simulink model "Lab1_Water_Tank_Level_Calibrated"  (R2017b)
settings: Solver=VariableStepAuto  StartTime=0.0  StopTime=60  RelTol=1e-3
settings Model: Creator=beena  LastModifiedBy=Joseph

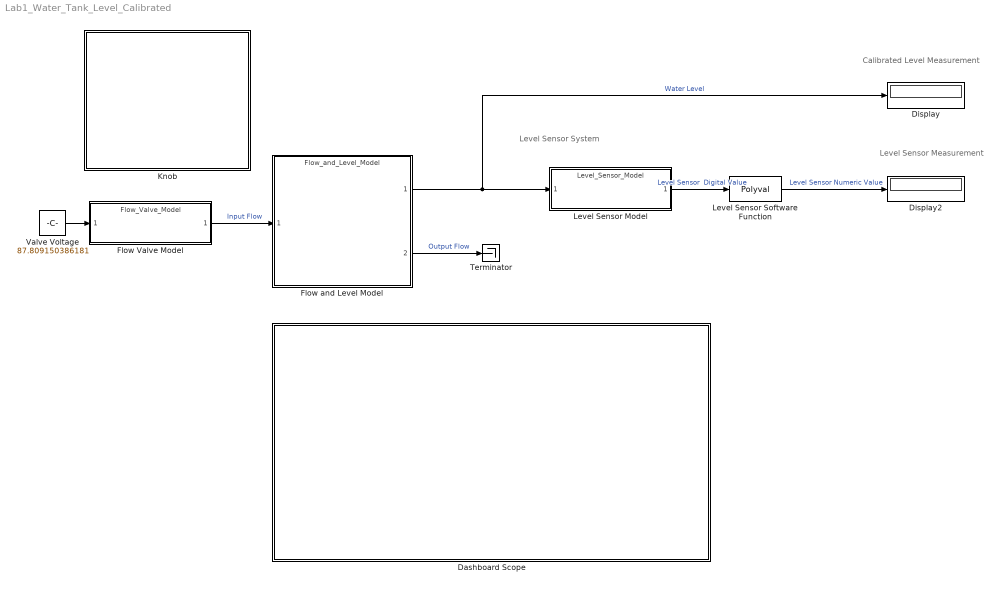
== system Lab1_Water_Tank_Level_Calibrated ==
  note: Level Sensor System
  note: Calibrated Level Measurement
  note: Level Sensor Measurement
  Dashboard Scope : Subsystem  DialogController=hmiCreateDDGDialog  IsWebBlock=on  mask(MWDashboardBlock){webBlockId=2a1a89e9-3606-4793-9b6e-01017e02ca12, webBlockType=sdiscope, ShowInitialText=on, HMISrcModelName=Lab1_Water_Tank_Level_Calibrated}
      mask prompts: webBlockId "WebBlock Id"; webBlockType "WebBlock Type"; HMISrcModelName "Source Model"
      mask help: SimulinkHMI:dialogs:HMIScopeDialogDesc
      mask Help: helpview([docroot '/mapfiles/simulink.map'], 'hmi_scope')
      mask Display:
      | if strcmp(get_param(bdroot(gcb),'BlockDiagramType'), 'library')
      |     image([(matlabroot) '/toolbox/simulink/hmi/icons/DashboardScope.png']);
      | end
  Display : Display
  Display2 : Display
  Flow Valve Model : ModelReference  ModelNameDialog=Flow_Valve_Model.slxp  ModelReferenceVersion=1.41  CopyOfModelProtected=on
  Flow and Level Model : ModelReference  ModelNameDialog=Flow_and_Level_Model.slxp  ModelReferenceVersion=1.41  CopyOfModelProtected=on
  Knob : Subsystem  DialogController=hmiCreateDDGDialog  IsWebBlock=on  mask(MWDashboardBlock){webBlockId=f1d15619-c2b9-4264-80fc-b36746c0ed4a, webBlockType=continuousknob, ShowInLibBrowser=on, ShowInitialText=on, HMISrcModelName=Lab1_Water_Tank_Level_Calibrated}
      mask prompts: webBlockId "WebBlock Id"; webBlockType "WebBlock Type"; HMISrcModelName "Source Model"
      mask help: SimulinkHMI:dialogs:ContinuousKnobDialogDesc
      mask Help: helpview([docroot '/mapfiles/simulink.map'], 'hmi_knob')
      mask Display:
      | if strcmp(get_param(bdroot(gcb),'BlockDiagramType'), 'library')
      |     image([(matlabroot) '/toolbox/simulink/hmi/icons/ContinuousKnob.png']);
      | end
  Level Sensor Software Function : Polyval  Coefs="[0.2001    0.0005]"
  Level Sensor Model : ModelReference  ModelNameDialog=Level_Sensor_Model.slxp  ModelReferenceVersion=1.51  CopyOfModelProtected=on
  Terminator : Terminator
  Valve Voltage : Constant  Value=87.809150386181
  wires:
  Flow and Level Model/1 -> Level Sensor Model/1, Display/1  "Water Level"
  Flow and Level Model/2 -> Terminator/1  "Output Flow"
  Flow Valve Model/1 -> Flow and Level Model/1  "Input Flow"
  Level Sensor Model/1 -> Level Sensor Software Function/1  "Level Sensor  Digital Value"
  Level Sensor Software Function/1 -> Display2/1  "Level Sensor Numeric Value"
  Valve Voltage/1 -> Flow Valve Model/1

== system Lab1_Water_Tank_Level_Calibrated/Dashboard Scope ==

== system Lab1_Water_Tank_Level_Calibrated/Knob ==
